simulink model "ec_fixed_slp_sb"  (Simulink 10.0)
settings: Solver=FixedStepDiscrete  StartTime=0.0  StopTime=10  RelTol=1e-3
PreLoadFcn:
  | ec_fixed_setup;
StartFcn:
  | tic;
StopFcn:
  | toc;
undefined symbols (not defined in the file): dfilt, ec_length, ec_lib, Fs, pic_frame_size, sm_length, Sources, spkr_to_mic_delay, spkr_to_mic_filter
libraries: dspsrcs4 x14, simulink x10, dspsigops x2, dspwin32 x2, dspbuff3 x1, dspobslib x1, dspsnks4 x1, dsparch4 x1
settings Model: Creator=Kerry Schutz  LastModifiedBy=bhisma
settings DataIOCC: LimitDataPoints=on  SignalLoggingSaveFormat=ModelDataLogs
settings OptimizationCC: BlockReduction=off  DefaultParameterBehavior=Inlined  InlineInvariantSignals=on  ExpressionDepthLimit=2147483647  StateBitsets=on  DataBitsets=on  ZeroExternalMemoryAtStartup=off  ZeroInternalMemoryAtStartup=off  EfficientFloat2IntCast=on  LifeSpan=1  EfficientTunableParamExpr=on
settings DebuggingCC: AlgebraicLoopMsg=none  SaveWithParameterizedLinksMsg=none  SolverPrmCheckMsg=warning  FcnCallInpInsideContextMsg=warning  StateNameClashWarn=warning
settings HardwareCC: ProdBitPerInt=16  ProdBitPerPointer=16  ProdBitPerSizeT=16  ProdBitPerPtrDiffT=16  ProdIntDivRoundTo=Zero  ProdEndianess=LittleEndian  ProdWordSize=16  ProdHWDeviceType=Microchip->dsPIC  TargetIntDivRoundTo=Zero  TargetEndianess=LittleEndian  TargetHWDeviceType=Microchip->dsPIC
settings SFSimCC: SimUseLocalCustomCode=on  SimParseCustomCode=off  MATLABDynamicMemAlloc=off  CustomCodeUndefinedFunction=FilterOut
settings RTWCC: Description=Real-Time Workshop Embedded Coder (no auto configuration)  SystemTargetFile=ert.tlc  GenCodeOnly=on  TemplateMakefile=ert_default_tmf  RTWUseLocalCustomCode=on
settings CodeAppCC: IgnoreCustomStorageClasses=off  CustomSymbolStrType=$N$R$M  InternalIdentifier=Classic  InlinedPrmAccess=Macros
settings ERTTargetCC: TargetFcnLib=ansi_tfl_tmw.mat  GenerateSampleERTMain=on  IncludeMdlTerminateFcn=off  SupportAbsoluteTime=off  PurelyIntegerCode=on  SupportNonFinite=off  SupportComplex=off  InlinedParameterPlacement=NonHierarchical  ERTCustomFileTemplate=example_file_process.tlc  ConvertIfToSwitch=off  SuppressUnreachableDefaultCases=off

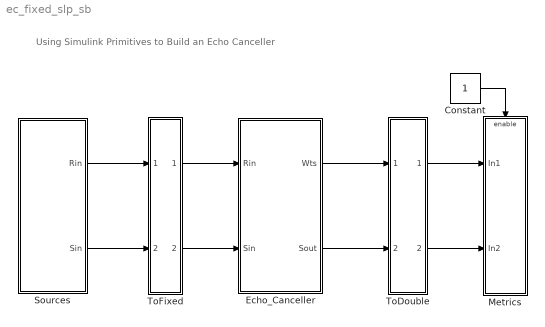
== system ec_fixed_slp_sb ==
  note: Using Simulink Primitives to Build an Echo Canceller
  Constant : Constant
  Echo_Canceller : Subsystem
  Metrics : Subsystem
  Sources : Subsystem  AncestorBlock=ec_lib/Sources
  ToDouble : Subsystem
  ToFixed : Subsystem
  wires:
  Sources/2(Sin) -> ToFixed/2(" In2")
  Sources/1(Rin) -> ToFixed/1(In1)
  ToDouble/2(Sout) -> Metrics/2(In2)
  ToDouble/1(Wts) -> Metrics/1(In1)
  Constant/1 -> Metrics/Enable
  ToFixed/1(Rin) -> Echo_Canceller/1(Rin)
  ToFixed/2(Sin) -> Echo_Canceller/2(Sin)
  Echo_Canceller/1(Wts) -> ToDouble/1(In1)
  Echo_Canceller/2(Sout) -> ToDouble/2(In2)

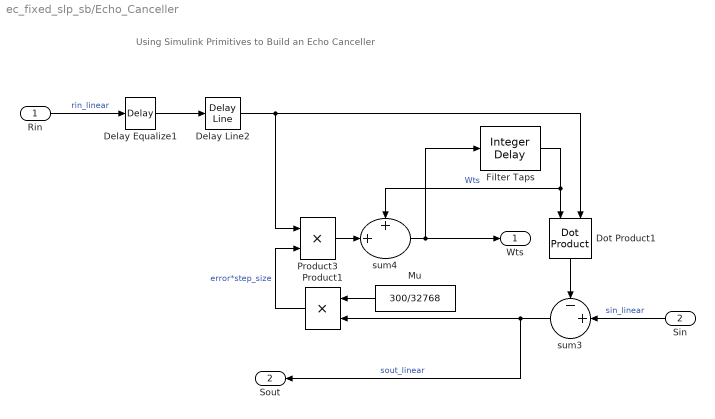
== system ec_fixed_slp_sb/Echo_Canceller ==
  note: Using Simulink Primitives to Build an Echo Canceller
  Rin : Inport
  Sin : Inport  Port=2
  Delay Equalize1 : dspsigops/Delay  dly_unit=Samples  delay=spkr_to_mic_delay +sm_length/2 - ec_length/2  ic_detail=off  dif_ic_for_ch=off  dif_ic_for_dly=off  ic=0  reset_popup=None
      settings: SourceProductName=DSP System Toolbox  SourceProductBaseCode=DS
  Delay Line2 : dspbuff3/Delay Line  siz=ec_length  ic=0  directfeed=on
      settings: SourceProductName=DSP System Toolbox  SourceProductBaseCode=DS
  Dot Product1 : simulink/Math Operations/Dot Product  OutDataTypeStr=fixdt(1,16,15)  OutputDataTypeScalingMode=Specify via dialog  OutDataType=fixdt(1,16,15)  OutScaling=[]  RndMeth=Nearest  DoSatur=off
      settings: SourceProductName=Simulink  SourceProductBaseCode=SL
  Filter Taps : dspobslib/Integer Delay  delay=ec_length  ic=0  reset_popup=None
      settings: SourceProductName=DSP System Toolbox  SourceProductBaseCode=DS
  Mu : Constant  Value=300/32768  OutDataTypeStr=fixdt(1,16,15)  SampleTime=pic_frame_size/Fs
  Product1 : Product  OutDataTypeStr=fixdt(1,16,15)  RndMeth=Nearest  SaturateOnIntegerOverflow=on
  Product3 : Product  OutDataTypeStr=fixdt(1,16,15)  RndMeth=Nearest  SaturateOnIntegerOverflow=on
  sum3 : Sum  Inputs=-+|  OutDataTypeStr=fixdt(1,16,14)  RndMeth=Nearest  SaturateOnIntegerOverflow=on
  sum4 : Sum  Inputs=++|  OutDataTypeStr=fixdt(1,16,15)  RndMeth=Nearest  SaturateOnIntegerOverflow=on
  Wts : Outport
  Sout : Outport  Port=2
  wires:
  Delay Equalize1/1 -> Delay Line2/1
  Filter Taps/1 -> sum4/1, Dot Product1/1  "Wts"
  sum4/1 -> Wts/1, Filter Taps/1
  Delay Line2/1 -> Dot Product1/2, Product3/1
  sum3/1 -> Product1/2, Sout/1  "sout_linear"
  Dot Product1/1 -> sum3/1
  Mu/1 -> Product1/1
  Product3/1 -> sum4/2
  Product1/1 -> Product3/2  "error*step_size"
  Rin/1 -> Delay Equalize1/1  "rin_linear"
  Sin/1 -> sum3/2  "sin_linear"

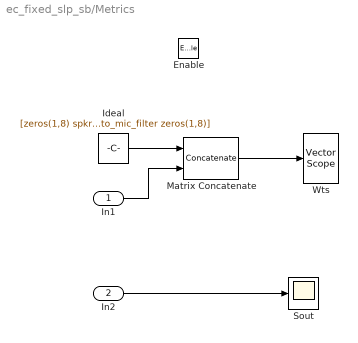
== system ec_fixed_slp_sb/Metrics ==
  In1 : Inport
  In2 : Inport  Port=2
  Enable : EnablePort
  Ideal : Constant  Value=[zeros(1,8) spkr_to_mic_filter zeros(1,8)]
  Matrix Concatenate : Concatenate  Mode=Multidimensional array  ConcatenateDimension=2
  Sout : Scope
  Wts : dspsnks4/Vector Scope  ScopeProperties=on  Domain=Time  HorizSpan=1  DisplayProperties=off  AxisGrid=on  Memory=off  FrameNumber=on  AxisLegend=off  AxisZoom=off  OpenScopeAtSimStart=on  OpenScopeImmediately=off  FigPos=[616 915 341 237]  AxisProperties=off  XUnits=Hertz  XRange=[0...Fs/2]  InheritXIncr=on  XIncr=1  XLabel=Time  XLimit=Auto  XMin=0  XMax=1  XStart=0  YUnits=dB  YLabel=Amplitude  LineProperties=off  LineColors=[1 0 0]|[0 1 0]
      settings: SourceProductName=DSP System Toolbox  SourceProductBaseCode=DS  YMin=-0.04794921875  YMax=0.335546875
  wires:
  In2/1 -> Sout/1
  Matrix Concatenate/1 -> Wts/1
  Ideal/1 -> Matrix Concatenate/1
  In1/1 -> Matrix Concatenate/2

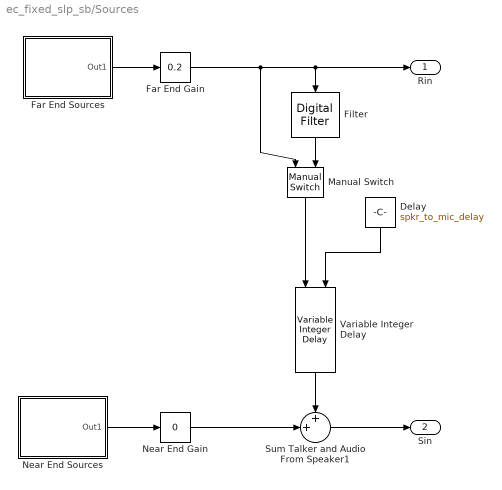
== system ec_fixed_slp_sb/Sources ==
  Delay : Constant  Value=spkr_to_mic_delay  SampleTime=1/Fs
  Far End Gain : simulink/Math Operations/Slider Gain  SystemSampleTime=-1  low=0  gain=0.2  high=10
  Far End Sources : Subsystem
  Filter : dsparch4/Digital Filter  Tag=BlockMethodSubSystem  TypePopup=FIR (all zeros)  IIRFiltStruct=Direct form II transposed  AllPoleFiltStruct=Direct form  FIRFiltStruct=Direct form  CoeffSource=Specify via dialog  NumCoeffs=spkr_to_mic_filter  DenCoeffs=[1 0.1]  BiQuadCoeffs=[1 0.3 0.4 1 0.1 0.2]  LatticeCoeffs=[0.2 0.4]  denIgnore=on  FiltPerSampPopup=One filter per frame  IC=0  ICnum=0  ICden=0  roundingMode=Floor  overflowMode=off  ScaleValues=1  scaleValueFracLength=14  stageInFracLength=15  stageOutFracLength=15  FilterSource=Specify via dialog  dfiltObjectName=dfilt.dffir([1 2 1])
      settings: SourceProductName=DSP System Toolbox  SourceProductBaseCode=DS
  Manual Switch : simulink/Signal Routing/Manual Switch  SystemSampleTime=-1  sw=0  action=0  varsize=off
      settings: SourceProductName=Simulink  SourceProductBaseCode=SL
  Near End Gain : simulink/Math Operations/Slider Gain  SystemSampleTime=-1  low=0  gain=0  high=10
  Near End Sources : Subsystem
  Sum Talker and Audio From Speaker1 : Sum  Inputs=++|  SaturateOnIntegerOverflow=on  InputSameDT=on  OutDataTypeStr=Inherit: Same as first input
  Variable Integer Delay : dspsigops/Variable Integer Delay  dmax=100  ic=0
      settings: SourceProductName=DSP System Toolbox  SourceProductBaseCode=DS
  Rin : Outport
  Sin : Outport  Port=2
  wires:
  Delay/1 -> Variable Integer Delay/2
  Manual Switch/1 -> Variable Integer Delay/1
  Variable Integer Delay/1 -> Sum Talker and Audio From Speaker1/1
  Sum Talker and Audio From Speaker1/1 -> Sin/1
  Filter/1 -> Manual Switch/2
  Far End Sources/1(Out1) -> Far End Gain/1
  Near End Sources/1(Out1) -> Near End Gain/1
  Near End Gain/1 -> Sum Talker and Audio From Speaker1/2
  Far End Gain/1 -> Manual Switch/1, Rin/1, Filter/1

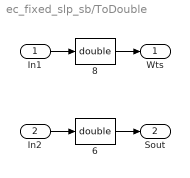
== system ec_fixed_slp_sb/ToDouble ==
  In1 : Inport
  In2 : Inport  Port=2
  " 6" : DataTypeConversion  OutDataTypeStr=double
  " 8" : DataTypeConversion  OutDataTypeStr=double
  Wts : Outport
  Sout : Outport  Port=2
  wires:
  In1/1 -> " 8"/1
  " 8"/1 -> Wts/1
  In2/1 -> " 6"/1
  " 6"/1 -> Sout/1

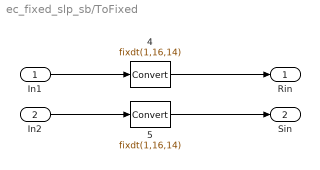
== system ec_fixed_slp_sb/ToFixed ==
  In1 : Inport
  " In2" : Inport  Port=2
  " 4" : DataTypeConversion  OutDataTypeStr=fixdt(1,16,14)
  " 5" : DataTypeConversion  OutDataTypeStr=fixdt(1,16,14)
  Rin : Outport
  Sin : Outport  Port=2
  wires:
  In1/1 -> " 4"/1
  " 4"/1 -> Rin/1
  " In2"/1 -> " 5"/1
  " 5"/1 -> Sin/1

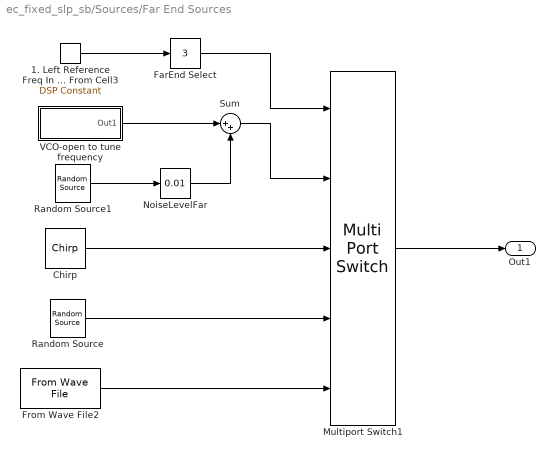
== system ec_fixed_slp_sb/Sources/Far End Sources ==
  1. Left Reference Freq In Hz From Cell3 : dspsrcs4/DSP Constant  SystemSampleTime=-1  Value=1  SampleMode=Discrete  discreteOutput=Sample-based  continuousOutput=Sample-based  sampTime=1/Fs  framePeriod=2  dataType=double  isSigned=on  wordLen=16  udDataType=sfix(16)  fracBitsMode=Best precision  numFracBits=15  InterpretAs1D=-inf  Ts=-inf  FramebasedOutput=-inf
      settings: SourceProductName=DSP System Toolbox  SourceProductBaseCode=DS  additionalParams=on
  Chirp : dspsrcs4/Chirp  sweep=Linear  mode=Unidirectional  f0=100  f1=4000  t1=pic_frame_size/Fs  Tsweep=pic_frame_size/Fs  phase=0  Ts=1/Fs  spf=1  datatype=Double
      settings: SourceProductName=DSP System Toolbox
  FarEnd Select : simulink/Math Operations/Slider Gain  SystemSampleTime=-1  low=0  gain=3  high=10
  From Wave File2 : dspwin32/From Wave File  FileName=far_end.wav  SamplesPerFrame=1  MinBufSize=80  dType=double  bLoop=on  timesToPlay=inf  restartMode=immediately after last sample  firstSampleOutput=off  lastSampleOutput=off
      settings: SourceProductName=DSP System Toolbox  SourceProductBaseCode=DS
  Multiport Switch1 : MultiPortSwitch  Inputs=4  SampleTime=1/Fs
  NoiseLevelFar : simulink/Math Operations/Slider Gain  SystemSampleTime=-1  low=0  gain=0.01  high=1
  Random Source : dspsrcs4/Random Source  SrcType=Gaussian  NormMethod=Ziggurat  CltLength=12  MinVal=0  MaxVal=1  MeanVal=0  VarVal=1  RepMode=Repeatable  rawSeed=1  IsInherit=off  SampMode=Discrete  SampTime=1/Fs  SampFrame=1  DataType=Double  OutComplex=Real
  Random Source1 : dspsrcs4/Random Source  SrcType=Gaussian  NormMethod=Ziggurat  CltLength=12  MinVal=0  MaxVal=1  MeanVal=0  VarVal=1  RepMode=Not repeatable  rawSeed=1  IsInherit=off  SampMode=Discrete  SampTime=1/Fs  SampFrame=1  DataType=Double  OutComplex=Real
  Sum : Sum  Inputs=|++
  VCO-open to tune frequency : Subsystem
  Out1 : Outport
  wires:
  NoiseLevelFar/1 -> Sum/2
  Random Source1/1 -> NoiseLevelFar/1
  Sum/1 -> Multiport Switch1/2
  FarEnd Select/1 -> Multiport Switch1/1
  1. Left Reference Freq In Hz From Cell3/1 -> FarEnd Select/1
  Random Source/1 -> Multiport Switch1/4
  Chirp/1 -> Multiport Switch1/3
  From Wave File2/1 -> Multiport Switch1/5
  Multiport Switch1/1 -> Out1/1
  VCO-open to tune frequency/1(Out1) -> Sum/1

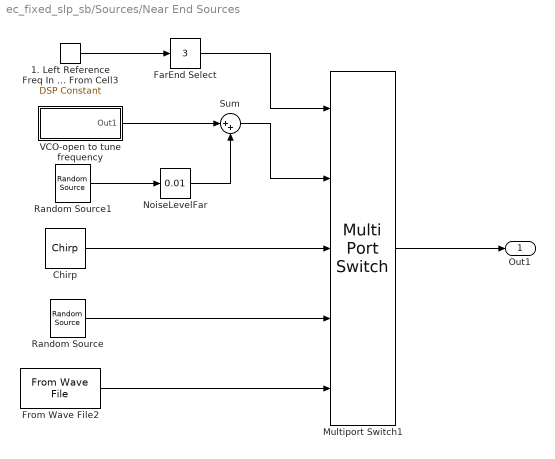
== system ec_fixed_slp_sb/Sources/Near End Sources ==
  1. Left Reference Freq In Hz From Cell3 : dspsrcs4/DSP Constant  SystemSampleTime=-1  Value=1  SampleMode=Discrete  discreteOutput=Sample-based  continuousOutput=Sample-based  sampTime=1/Fs  framePeriod=2  dataType=double  isSigned=on  wordLen=16  udDataType=sfix(16)  fracBitsMode=Best precision  numFracBits=15  InterpretAs1D=-inf  Ts=-inf  FramebasedOutput=-inf
      settings: SourceProductName=DSP System Toolbox  SourceProductBaseCode=DS  additionalParams=on
  Chirp : dspsrcs4/Chirp  sweep=Linear  mode=Unidirectional  f0=100  f1=4000  t1=pic_frame_size/Fs  Tsweep=pic_frame_size/Fs  phase=0  Ts=1/Fs  spf=1  datatype=Double
      settings: SourceProductName=DSP System Toolbox
  FarEnd Select : simulink/Math Operations/Slider Gain  SystemSampleTime=-1  low=0  gain=3  high=10
  From Wave File2 : dspwin32/From Wave File  FileName=far_end.wav  SamplesPerFrame=1  MinBufSize=80  dType=double  bLoop=on  timesToPlay=inf  restartMode=immediately after last sample  firstSampleOutput=off  lastSampleOutput=off
      settings: SourceProductName=DSP System Toolbox  SourceProductBaseCode=DS
  Multiport Switch1 : MultiPortSwitch  Inputs=4  SampleTime=1/Fs
  NoiseLevelFar : simulink/Math Operations/Slider Gain  SystemSampleTime=-1  low=0  gain=0.01  high=1
  Random Source : dspsrcs4/Random Source  SrcType=Gaussian  NormMethod=Ziggurat  CltLength=12  MinVal=0  MaxVal=1  MeanVal=0  VarVal=1  RepMode=Repeatable  rawSeed=1  IsInherit=off  SampMode=Discrete  SampTime=1/Fs  SampFrame=1  DataType=Double  OutComplex=Real
  Random Source1 : dspsrcs4/Random Source  SrcType=Gaussian  NormMethod=Ziggurat  CltLength=12  MinVal=0  MaxVal=1  MeanVal=0  VarVal=1  RepMode=Not repeatable  rawSeed=1  IsInherit=off  SampMode=Discrete  SampTime=1/Fs  SampFrame=1  DataType=Double  OutComplex=Real
  Sum : Sum  Inputs=|++
  VCO-open to tune frequency : Subsystem
  Out1 : Outport
  wires:
  VCO-open to tune frequency/1(Out1) -> Sum/1
  Multiport Switch1/1 -> Out1/1
  From Wave File2/1 -> Multiport Switch1/5
  Chirp/1 -> Multiport Switch1/3
  Random Source/1 -> Multiport Switch1/4
  1. Left Reference Freq In Hz From Cell3/1 -> FarEnd Select/1
  FarEnd Select/1 -> Multiport Switch1/1
  Sum/1 -> Multiport Switch1/2
  Random Source1/1 -> NoiseLevelFar/1
  NoiseLevelFar/1 -> Sum/2

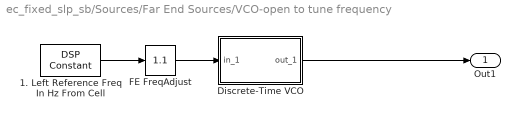
== system ec_fixed_slp_sb/Sources/Far End Sources/VCO-open to tune frequency ==
  1. Left Reference Freq In Hz From Cell : dspsrcs4/DSP Constant  SystemSampleTime=-1  Value=1000  SampleMode=Discrete  discreteOutput=Sample-based  continuousOutput=Sample-based  sampTime=1/Fs  framePeriod=2  dataType=double  isSigned=on  wordLen=16  udDataType=sfix(16)  fracBitsMode=Best precision  numFracBits=15  InterpretAs1D=-inf  Ts=-inf  FramebasedOutput=-inf
      settings: SourceProductName=DSP System Toolbox  SourceProductBaseCode=DS  additionalParams=on
  Discrete-Time VCO : Subsystem  mask(Discrete-Time VCO){Ac=1, Fc=0, Kc=1, Ph=pi/2, ts=1/Fs}
      mask prompts: Ac "Output amplitude:"; Fc "Oscillation frequency (Hz):"; Kc "Input sensitivity:"; Ph "Initial phase (rad):"; ts "Sample time:"
      mask help: Generate a discrete-time output signal whose frequency changes in response to the amplitude variations of the input signal. The input signal must be a scalar.
      mask init:
      | if ((length(Ac)~=1) | (length(Fc)~=1) | (length(Kc)~=1) | (length(Ph)~=1) | (length(ts)~=1) |(length(Ph)~=1))error('Mask parameters must be scalar values.');end;
      | pi2=2*pi;
      mask Help: helpview(commbhelp)
      mask Display: disp('Discrete-Time\nVCO (rab)')
  FE FreqAdjust : simulink/Math Operations/Slider Gain  SystemSampleTime=-1  low=0  gain=1.1  high=5
  Out1 : Outport
  wires:
  1. Left Reference Freq In Hz From Cell/1 -> FE FreqAdjust/1
  FE FreqAdjust/1 -> Discrete-Time VCO/1(in_1)
  Discrete-Time VCO/1(out_1) -> Out1/1

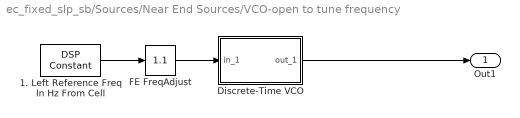
== system ec_fixed_slp_sb/Sources/Near End Sources/VCO-open to tune frequency ==
  1. Left Reference Freq In Hz From Cell : dspsrcs4/DSP Constant  SystemSampleTime=-1  Value=1000  SampleMode=Discrete  discreteOutput=Sample-based  continuousOutput=Sample-based  sampTime=1/Fs  framePeriod=2  dataType=double  isSigned=on  wordLen=16  udDataType=sfix(16)  fracBitsMode=Best precision  numFracBits=15  InterpretAs1D=-inf  Ts=-inf  FramebasedOutput=-inf
      settings: SourceProductName=DSP System Toolbox  SourceProductBaseCode=DS  additionalParams=on
  Discrete-Time VCO : Subsystem  mask(Discrete-Time VCO){Ac=1, Fc=0, Kc=1, Ph=pi/2, ts=1/Fs}
      mask prompts: Ac "Output amplitude:"; Fc "Oscillation frequency (Hz):"; Kc "Input sensitivity:"; Ph "Initial phase (rad):"; ts "Sample time:"
      mask help: Generate a discrete-time output signal whose frequency changes in response to the amplitude variations of the input signal. The input signal must be a scalar.
      mask init:
      | if ((length(Ac)~=1) | (length(Fc)~=1) | (length(Kc)~=1) | (length(Ph)~=1) | (length(ts)~=1) |(length(Ph)~=1))error('Mask parameters must be scalar values.');end;
      | pi2=2*pi;
      mask Help: helpview(commbhelp)
      mask Display: disp('Discrete-Time\nVCO (rab)')
  FE FreqAdjust : simulink/Math Operations/Slider Gain  SystemSampleTime=-1  low=0  gain=1.1  high=5
  Out1 : Outport
  wires:
  Discrete-Time VCO/1(out_1) -> Out1/1
  FE FreqAdjust/1 -> Discrete-Time VCO/1(in_1)
  1. Left Reference Freq In Hz From Cell/1 -> FE FreqAdjust/1

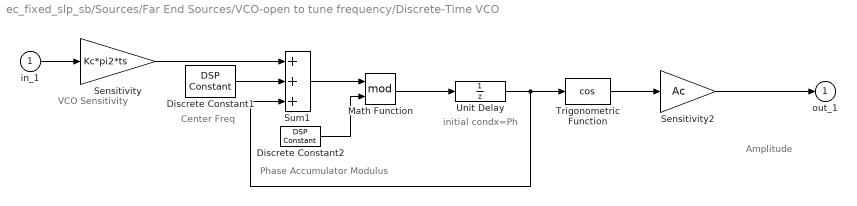
== system ec_fixed_slp_sb/Sources/Far End Sources/VCO-open to tune frequency/Discrete-Time VCO ==
  note: initial condx=Ph
  note: VCO Sensitivity
  note: Center Freq
  note: Phase Accumulator
      | Modulus
  note: Amplitude
  in_1 : Inport
  Discrete Constant1 : dspsrcs4/DSP Constant  SystemSampleTime=-1  Value=Fc*pi2*ts  SampleMode=Discrete  discreteOutput=Sample-based (interpret vectors as 1-D)  continuousOutput=Sample-based  sampTime=1/8000  framePeriod=1/8000  dataType=Inherit via back propagation  isSigned=on  wordLen=16  udDataType=sfix(16)  fracBitsMode=Best precision  numFracBits=15  InterpretAs1D=on  Ts=1/8000  FramebasedOutput=off
      settings: SourceProductName=DSP System Toolbox  SourceProductBaseCode=DS  additionalParams=on
  Discrete Constant2 : dspsrcs4/DSP Constant  SystemSampleTime=-1  Value=pi2  SampleMode=Discrete  discreteOutput=Sample-based (interpret vectors as 1-D)  continuousOutput=Sample-based  sampTime=1/8000  framePeriod=1/8000  dataType=Inherit via back propagation  isSigned=on  wordLen=16  udDataType=sfix(16)  fracBitsMode=Best precision  numFracBits=15  InterpretAs1D=on  Ts=1/8000  FramebasedOutput=off
      settings: SourceProductName=DSP System Toolbox  SourceProductBaseCode=DS  additionalParams=on
  Math Function : Math  Operator=mod  SaturateOnIntegerOverflow=on
  Sensitivity : Gain  Gain=Kc*pi2*ts  SaturateOnIntegerOverflow=on  OutDataTypeStr=Inherit: Same as input  ParamDataTypeStr=Inherit: Same as input
  Sensitivity2 : Gain  Gain=Ac  SaturateOnIntegerOverflow=on  OutDataTypeStr=Inherit: Same as input  ParamDataTypeStr=Inherit: Same as input
  Sum1 : Sum  Inputs=+++  SaturateOnIntegerOverflow=on  InputSameDT=on  OutDataTypeStr=Inherit: Same as first input
  Trigonometric Function : Trigonometry  Operator=cos
  Unit Delay : UnitDelay  InitialCondition=Ph  SampleTime=ts
  out_1 : Outport  InitialOutput=0
  wires:
  Discrete Constant2/1 -> Math Function/2
  Sum1/1 -> Math Function/1
  Math Function/1 -> Unit Delay/1
  in_1/1 -> Sensitivity/1
  Sensitivity/1 -> Sum1/1
  Unit Delay/1 -> Sum1/3, Trigonometric Function/1
  Trigonometric Function/1 -> Sensitivity2/1
  Sensitivity2/1 -> out_1/1
  Discrete Constant1/1 -> Sum1/2

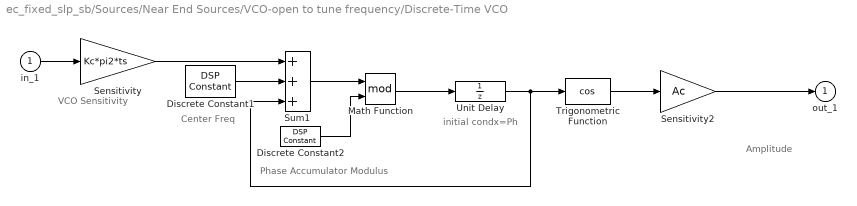
== system ec_fixed_slp_sb/Sources/Near End Sources/VCO-open to tune frequency/Discrete-Time VCO ==
  note: Amplitude
  note: Phase Accumulator
      | Modulus
  note: Center Freq
  note: VCO Sensitivity
  note: initial condx=Ph
  in_1 : Inport
  Discrete Constant1 : dspsrcs4/DSP Constant  SystemSampleTime=-1  Value=Fc*pi2*ts  SampleMode=Discrete  discreteOutput=Sample-based (interpret vectors as 1-D)  continuousOutput=Sample-based  sampTime=1/8000  framePeriod=1/8000  dataType=Inherit via back propagation  isSigned=on  wordLen=16  udDataType=sfix(16)  fracBitsMode=Best precision  numFracBits=15  InterpretAs1D=on  Ts=1/8000  FramebasedOutput=off
      settings: SourceProductName=DSP System Toolbox  SourceProductBaseCode=DS  additionalParams=on
  Discrete Constant2 : dspsrcs4/DSP Constant  SystemSampleTime=-1  Value=pi2  SampleMode=Discrete  discreteOutput=Sample-based (interpret vectors as 1-D)  continuousOutput=Sample-based  sampTime=1/8000  framePeriod=1/8000  dataType=Inherit via back propagation  isSigned=on  wordLen=16  udDataType=sfix(16)  fracBitsMode=Best precision  numFracBits=15  InterpretAs1D=on  Ts=1/8000  FramebasedOutput=off
      settings: SourceProductName=DSP System Toolbox  SourceProductBaseCode=DS  additionalParams=on
  Math Function : Math  Operator=mod  SaturateOnIntegerOverflow=on
  Sensitivity : Gain  Gain=Kc*pi2*ts  SaturateOnIntegerOverflow=on  OutDataTypeStr=Inherit: Same as input  ParamDataTypeStr=Inherit: Same as input
  Sensitivity2 : Gain  Gain=Ac  SaturateOnIntegerOverflow=on  OutDataTypeStr=Inherit: Same as input  ParamDataTypeStr=Inherit: Same as input
  Sum1 : Sum  Inputs=+++  SaturateOnIntegerOverflow=on  InputSameDT=on  OutDataTypeStr=Inherit: Same as first input
  Trigonometric Function : Trigonometry  Operator=cos
  Unit Delay : UnitDelay  InitialCondition=Ph  SampleTime=ts
  out_1 : Outport  InitialOutput=0
  wires:
  Discrete Constant1/1 -> Sum1/2
  Sensitivity2/1 -> out_1/1
  Trigonometric Function/1 -> Sensitivity2/1
  Unit Delay/1 -> Trigonometric Function/1, Sum1/3
  Sensitivity/1 -> Sum1/1
  in_1/1 -> Sensitivity/1
  Math Function/1 -> Unit Delay/1
  Sum1/1 -> Math Function/1
  Discrete Constant2/1 -> Math Function/2
